simulink model "simplifiedManipulatorModel"  (R2020b)
settings: Solver=VariableStepAuto  StartTime=0.0  StopTime=10.0  RelTol=1e-3
PreLoadFcn:
  | initModelData
values from neighbouring files (symbols this model uses):
  B = Bm + (Kb*Km)/R    (= 0.0149065789474)    [initModelData.m]
  Jm = 6.1e-4    (= 0.00061)    [initModelData.m]
  Km = 0.105    [initModelData.m]
  R = 0.76    [initModelData.m]
settings Model: Creator=esdan  LastModifiedBy=esdan

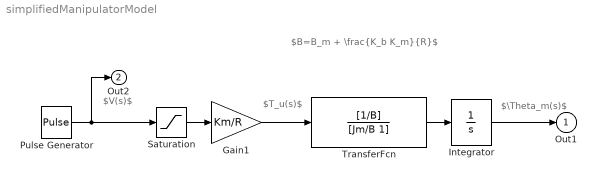
== system simplifiedManipulatorModel ==
  note: $\Theta_m(s)$
  note: $V(s)$
  note: $T_u(s)$
  note: $B=B_m + \frac{K_b K_m}{R}$
  Gain1 : Gain  Gain=Km/R
  Integrator : Integrator
  Pulse Generator : DiscretePulseGenerator  PulseType=Time based  Period=10  PulseWidth=33
  Saturation : Saturate  UpperLimit=35  LowerLimit=-35
  TransferFcn : TransferFcn  Numerator=[1/B]  Denominator=[Jm/B 1]
  Out1 : Outport  SignalName=posSimplified
  Out2 : Outport  Port=2  SignalName=V
  wires:
  Pulse Generator/1 -> Saturation/1, Out2/1
  TransferFcn/1 -> Integrator/1
  Gain1/1 -> TransferFcn/1
  Integrator/1 -> Out1/1
  Saturation/1 -> Gain1/1
